simulink model "HW2_PR2"  (R2019a)
settings: Solver=VariableStepAuto  StartTime=0.0  StopTime=1500  RelTol=1e-3
InitFcn:
  | MKM506E_HW2_Q2_parameters
values from neighbouring files (symbols this model uses):
  b = 20    [HW2_P2_a.m]    (also in HW2_Q2_parameters.m)
  k_1 = 25    [HW2_P2_a.m]    (also in HW2_Q2_parameters.m)
  k_2 = 12    [HW2_P2_a.m]    (also in HW2_Q2_parameters.m)
  m_1 = 100    [HW2_P2_a.m]    (also in HW2_Q2_parameters.m)
  m_2 = 500    [HW2_P2_a.m]    (also in HW2_Q2_parameters.m)
settings Model: Creator=canba  LastModifiedBy=canba

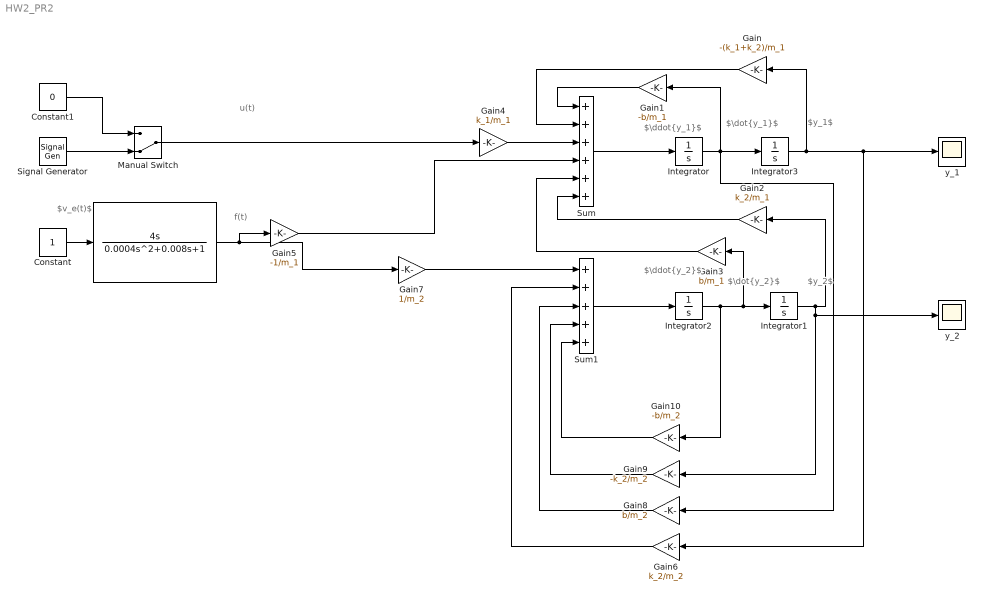
== system HW2_PR2 ==
  note: $v_e(t)$
  note: f(t)
  note: u(t)
  note: $y_2$
  note: $y_1$
  note: $\dot{y_1}$
  note: $\dot{y_2}$
  note: $\ddot{y_1}$
  note: $\ddot{y_2}$
  " " : TransferFcn  Numerator=[4 0]  Denominator=[0.0004 0.008 1]
  Constant : Constant
  Constant1 : Constant  Value=0
  Gain : Gain  Gain=-(k_1+k_2)/m_1
  Gain1 : Gain  Gain=-b/m_1
  Gain10 : Gain  Gain=-b/m_2
  Gain2 : Gain  Gain=k_2/m_1
  Gain3 : Gain  Gain=b/m_1
  Gain4 : Gain  Gain=k_1/m_1
  Gain5 : Gain  Gain=-1/m_1
  Gain6 : Gain  Gain=k_2/m_2
  Gain7 : Gain  Gain=1/m_2
  Gain8 : Gain  Gain=b/m_2
  Gain9 : Gain  Gain=-k_2/m_2
  Integrator{,1..3} (4 alike) : Integrator
  Manual Switch : ManualSwitch  CurrentSetting=0
  Signal Generator : SignalGenerator  WaveForm=square  Frequency=0.002
  Sum : Sum  Inputs=6
  Sum1 : Sum  Inputs=5
  y_1 : Scope
  "y_2 " : Scope
  wires:
  Integrator/1 -> Gain8/1, Integrator3/1, Gain1/1
  Integrator2/1 -> Gain3/1, Integrator1/1, Gain10/1
  Sum/1 -> Integrator/1
  Integrator3/1 -> y_1/1, Gain6/1, Gain/1
  Integrator1/1 -> Gain9/1, "y_2 "/1, Gain2/1
  Sum1/1 -> Integrator2/1
  Gain1/1 -> Sum/1
  Gain/1 -> Sum/2
  Gain2/1 -> Sum/6
  Gain3/1 -> Sum/5
  Gain4/1 -> Sum/3
  Gain5/1 -> Sum/4
  " "/1 -> Gain5/1, Gain7/1
  Gain7/1 -> Sum1/1
  Gain6/1 -> Sum1/2
  Gain8/1 -> Sum1/3
  Gain9/1 -> Sum1/4
  Gain10/1 -> Sum1/5
  Constant1/1 -> Manual Switch/1
  Signal Generator/1 -> Manual Switch/2
  Manual Switch/1 -> Gain4/1
  Constant/1 -> " "/1
